simulink model "Simulations"  (R2020b)
settings: Solver=VariableStepAuto  StartTime=0.0  StopTime=100  MinStep=0.0001  RelTol=1e-3
undefined symbols (not defined in the file or in its folder): chassis, FTP, powertrain, sigbuilder_block
libraries: sdl_lib x364, nesl_utility x336, fl_lib x224, aerolibconvert2 x28, pid_lib x27
(part 14 of 15)

== system Simulations/Plant Model7 ==
  note: Chassis
  note: Motor Dynamics
  note: Drivetrain
  trq_cmd : Inport
  road_grade : Inport  Port=2
  Angle Conversion3 : aerolibconvert2/Angle Conversion  IU=deg  OU=rad
  Belt Drive FL : sdl_lib/Couplings & Drives/Belt Drive  drive_type=sdl.enum.wrap_configuration.open  belt_type=sdl.enum.belt_type.ideal  sheave_ang=30 deg  num_belts=1  model_f_c=sdl.enum.model_centrifugal.off  linear_density=0.6 kg/m  model_compliance=sdl.enum.compliance.off  stiffness=1e4 N/m  damping=1e3 N/(m/s)  tension=100 N  breakable=sdl.enum.max_tension.off  F_max=1e5 N  r_pulley_A=drivetrain.RadiusA m  r_pulley_B=drivetrain.RadiusB m  b_pulley_A=drivetrain.bvfCoeffA N*m/(rad/s)  b_pulley_B=drivetrain.bvfCoeffB N*m/(rad/s)  model_inertia_A=sdl.enum.model_inertia.off  model_inertia_B=sdl.enum.model_inertia.off  pulley_inertia_A=0.01 kg*m^2  pulley_inertia_B=0.03 kg*m^2  initial_velocity_A=0 rad/s  initial_velocity_B=0 rad/s  mu=0.5  wrap_parameterization=sdl.enum.wrap_parameterization.centers  d_centers=0.5 m  phi_wrap_A=145 deg  phi_wrap_B=215 deg  v_thr=0.001 m/s
      settings: SourceProductBaseCode=LD  InternalSimscapePortConfiguration="{\"Bottom\":[],\"Left\":[{\"id\":\"A\",\"label\":\"A\",\"type\":\"foundation.mechanical.rotational.rotational\"}],\"Right\":[{\"id\":\"B\",\"label\":\"B\",\"type\":\"foundation.mechanical.rotational.rotational\"}],\"Top\":[]}"
  Belt Drive FR : sdl_lib/Couplings & Drives/Belt Drive  drive_type=sdl.enum.wrap_configuration.open  belt_type=sdl.enum.belt_type.ideal  sheave_ang=30 deg  num_belts=1  model_f_c=sdl.enum.model_centrifugal.off  linear_density=0.6 kg/m  model_compliance=sdl.enum.compliance.off  stiffness=1e4 N/m  damping=1e3 N/(m/s)  tension=100 N  breakable=sdl.enum.max_tension.off  F_max=1e5 N  r_pulley_A=drivetrain.RadiusA m  r_pulley_B=drivetrain.RadiusB m  b_pulley_A=drivetrain.bvfCoeffA N*m/(rad/s)  b_pulley_B=drivetrain.bvfCoeffB N*m/(rad/s)  model_inertia_A=sdl.enum.model_inertia.off  model_inertia_B=sdl.enum.model_inertia.off  pulley_inertia_A=0.01 kg*m^2  pulley_inertia_B=0.03 kg*m^2  initial_velocity_A=0 rad/s  initial_velocity_B=0 rad/s  mu=0.5  wrap_parameterization=sdl.enum.wrap_parameterization.centers  d_centers=0.5 m  phi_wrap_A=145 deg  phi_wrap_B=215 deg  v_thr=0.001 m/s
      settings: SourceProductBaseCode=LD  InternalSimscapePortConfiguration="{\"Bottom\":[],\"Left\":[{\"id\":\"A\",\"label\":\"A\",\"type\":\"foundation.mechanical.rotational.rotational\"}],\"Right\":[{\"id\":\"B\",\"label\":\"B\",\"type\":\"foundation.mechanical.rotational.rotational\"}],\"Top\":[]}"
  Belt Drive RL : sdl_lib/Couplings & Drives/Belt Drive  drive_type=sdl.enum.wrap_configuration.open  belt_type=sdl.enum.belt_type.ideal  sheave_ang=30 deg  num_belts=1  model_f_c=sdl.enum.model_centrifugal.off  linear_density=0.6 kg/m  model_compliance=sdl.enum.compliance.off  stiffness=1e4 N/m  damping=1e3 N/(m/s)  tension=100 N  breakable=sdl.enum.max_tension.off  F_max=1e5 N  r_pulley_A=drivetrain.RadiusA m  r_pulley_B=drivetrain.RadiusB m  b_pulley_A=drivetrain.bvfCoeffA N*m/(rad/s)  b_pulley_B=drivetrain.bvfCoeffB N*m/(rad/s)  model_inertia_A=sdl.enum.model_inertia.off  model_inertia_B=sdl.enum.model_inertia.off  pulley_inertia_A=0.01 kg*m^2  pulley_inertia_B=0.03 kg*m^2  initial_velocity_A=0 rad/s  initial_velocity_B=0 rad/s  mu=0.5  wrap_parameterization=sdl.enum.wrap_parameterization.centers  d_centers=0.5 m  phi_wrap_A=145 deg  phi_wrap_B=215 deg  v_thr=0.001 m/s
      settings: SourceProductBaseCode=LD  InternalSimscapePortConfiguration="{\"Bottom\":[],\"Left\":[{\"id\":\"A\",\"label\":\"A\",\"type\":\"foundation.mechanical.rotational.rotational\"}],\"Right\":[{\"id\":\"B\",\"label\":\"B\",\"type\":\"foundation.mechanical.rotational.rotational\"}],\"Top\":[]}"
  Belt Drive RR : sdl_lib/Couplings & Drives/Belt Drive  drive_type=sdl.enum.wrap_configuration.open  belt_type=sdl.enum.belt_type.ideal  sheave_ang=30 deg  num_belts=1  model_f_c=sdl.enum.model_centrifugal.off  linear_density=0.6 kg/m  model_compliance=sdl.enum.compliance.off  stiffness=1e4 N/m  damping=1e3 N/(m/s)  tension=100 N  breakable=sdl.enum.max_tension.off  F_max=1e5 N  r_pulley_A=drivetrain.RadiusA m  r_pulley_B=drivetrain.RadiusB m  b_pulley_A=drivetrain.bvfCoeffA N*m/(rad/s)  b_pulley_B=drivetrain.bvfCoeffB N*m/(rad/s)  model_inertia_A=sdl.enum.model_inertia.off  model_inertia_B=sdl.enum.model_inertia.off  pulley_inertia_A=0.01 kg*m^2  pulley_inertia_B=0.03 kg*m^2  initial_velocity_A=0 rad/s  initial_velocity_B=0 rad/s  mu=0.5  wrap_parameterization=sdl.enum.wrap_parameterization.centers  d_centers=0.5 m  phi_wrap_A=145 deg  phi_wrap_B=215 deg  v_thr=0.001 m/s
      settings: SourceProductBaseCode=LD  InternalSimscapePortConfiguration="{\"Bottom\":[],\"Left\":[{\"id\":\"A\",\"label\":\"A\",\"type\":\"foundation.mechanical.rotational.rotational\"}],\"Right\":[{\"id\":\"B\",\"label\":\"B\",\"type\":\"foundation.mechanical.rotational.rotational\"}],\"Top\":[]}"
  Constant : Constant  Value=0
  Ideal Torque Source FL : fl_lib/Mechanical/Mechanical Sources/Ideal Torque Source
  Ideal Torque Source FR : fl_lib/Mechanical/Mechanical Sources/Ideal Torque Source
  Ideal Torque Source RL : fl_lib/Mechanical/Mechanical Sources/Ideal Torque Source
  Ideal Torque Source RR : fl_lib/Mechanical/Mechanical Sources/Ideal Torque Source
  Mechanical Rotational Reference{1..3,8} (4 alike) : fl_lib/Mechanical/Rotational Elements/Mechanical Rotational Reference
  Motor Delay : TransferFcn  Numerator=[0.01]  Denominator=[0.005 0.06 0.1001]
  PS-Simulink Converter{,1,3..4} (4 alike) : nesl_utility/PS-Simulink Converter  PhysicalDomain=network_engine_domain  SubClassName=ps_output  LeftPortType=input  RightPortType=output  PseudoPeriodic=off  Frequencies=[]  Unit=inherit  AffineConversion=off
  Simulink-PS Converter{3,9..12} (5 alike) : nesl_utility/Simulink-PS Converter  PhysicalDomain=network_engine_domain  SubClassName=ps_input  LeftPortType=input  RightPortType=output  PseudoPeriodic=off  Frequencies=[]  NoiseDistribution=none  NoiseParameters=[]  Unit=1  AffineConversion=off  FilteringAndDerivatives=provide  SimscapeFilterOrder=1  InputFilterTimeConstant=0.001  UdotUserProvided=0
  Simulink-PS Converter8 : nesl_utility/Simulink-PS Converter  PhysicalDomain=network_engine_domain  SubClassName=ps_input  LeftPortType=input  RightPortType=output  PseudoPeriodic=off  Frequencies=[]  NoiseDistribution=none  NoiseParameters=[]  Unit=rad  AffineConversion=off  FilteringAndDerivatives=provide  SimscapeFilterOrder=1  InputFilterTimeConstant=0.001  UdotUserProvided=0
  Solver Configuration2 : nesl_utility/Solver Configuration  PhysicalDomain=network_engine_domain  SubClassName=solver  LeftPortType=input  RightPortType=generic  Tones=[]  Harmonics=[]  SimulateNoise=off  Profile=off  UseLocalSampling=off  EnableSwitchedLinearOptims=on  FrequencyDomain=off  UseCCode=off  RelTol=0.001  AbsTol=1e-06  MinStep=1e-09  ToWorkspace=off  RevertToSquareIcSolve=off  NumHomotopyIterations=100  PhasorMode=off  PhasorModeNumHarmonics=1  DoDC=off  ResidualTolerance=1e-09  UseLocalSolver=off  LocalSolverChoice=NE_BACKWARD_EULER_ADVANCER  LocalSolverSampleTime=0.001  DoFixedCost=off  MaxNonlinIter=3  MaxModeIter=2  ComputeImpulses=off  ImpulseIterations=2  LinearAlgebra=auto  EquationFormulation=NE_TIME_EF  DelaysMemoryBudget=1024  AutomaticFiltering=on  FilteringTimeConstant=0.001  PartitionStorageMethod=AS_NEEDED  PartitionMemoryBudget=1024  PartitionMethod=ROBUST
  Terminator{,1..3} (4 alike) : Terminator
  Tire (Simple) FL : sdl_lib/Tires & Vehicles/Tire (Simple)  r_tire=drivetrain.RolRadius m  model_compliance=0  stiffness=1e6 N/m  damping=1000 N/(m/s)  model_inertia=0  tire_inertia=drivetrain.IyyWhl kg*m^2  initial_velocity=drivetrain.InitVelo rad/s
      settings: SourceProductBaseCode=LD  InternalSimscapePortConfiguration="{\"Bottom\":[],\"Left\":[{\"id\":\"A\",\"label\":\"A\",\"type\":\"foundation.mechanical.rotational.rotational\"}],\"Right\":[{\"id\":\"H\",\"label\":\"H\",\"type\":\"foundation.mechanical.translational.translational\"}],\"Top\":[]}"
  Tire (Simple) FR : sdl_lib/Tires & Vehicles/Tire (Simple)  r_tire=drivetrain.RolRadius m  model_compliance=0  stiffness=1e6 N/m  damping=1000 N/(m/s)  model_inertia=0  tire_inertia=drivetrain.IyyWhl kg*m^2  initial_velocity=drivetrain.InitVelo rad/s
      settings: SourceProductBaseCode=LD  InternalSimscapePortConfiguration="{\"Bottom\":[],\"Left\":[{\"id\":\"A\",\"label\":\"A\",\"type\":\"foundation.mechanical.rotational.rotational\"}],\"Right\":[{\"id\":\"H\",\"label\":\"H\",\"type\":\"foundation.mechanical.translational.translational\"}],\"Top\":[]}"
  Tire (Simple) RL : sdl_lib/Tires & Vehicles/Tire (Simple)  r_tire=drivetrain.RolRadius m  model_compliance=0  stiffness=1e6 N/m  damping=1000 N/(m/s)  model_inertia=0  tire_inertia=drivetrain.IyyWhl kg*m^2  initial_velocity=drivetrain.InitVelo rad/s
      settings: SourceProductBaseCode=LD  InternalSimscapePortConfiguration="{\"Bottom\":[],\"Left\":[{\"id\":\"A\",\"label\":\"A\",\"type\":\"foundation.mechanical.rotational.rotational\"}],\"Right\":[{\"id\":\"H\",\"label\":\"H\",\"type\":\"foundation.mechanical.translational.translational\"}],\"Top\":[]}"
  Tire (Simple) RR : sdl_lib/Tires & Vehicles/Tire (Simple)  r_tire=drivetrain.RolRadius m  model_compliance=0  stiffness=1e6 N/m  damping=1000 N/(m/s)  model_inertia=0  tire_inertia=drivetrain.IyyWhl kg*m^2  initial_velocity=drivetrain.InitVelo rad/s
      settings: SourceProductBaseCode=LD  InternalSimscapePortConfiguration="{\"Bottom\":[],\"Left\":[{\"id\":\"A\",\"label\":\"A\",\"type\":\"foundation.mechanical.rotational.rotational\"}],\"Right\":[{\"id\":\"H\",\"label\":\"H\",\"type\":\"foundation.mechanical.translational.translational\"}],\"Top\":[]}"
  Tire-Road Interaction (Magic Formula) FL : sdl_lib/Tires & Vehicles/Tire Subcomponents/Tire-Road Interaction (Magic Formula)  parameterization=sdl.enum.magic_tire_model.peak  F_z1=drivetrain.VertLoad N  F_x1=drivetrain.PeakLongF N  kappa1=drivetrain.Slip  B_m=10  C_m=1.9  D_m=1  E_m=0.97  fz0=4000 N  p_Cx=1.685  p_Dx=[1.21, -.037]  p_Ex=[.344, .095, -.02, 0]  p_Kx=[21.51, -.163, .245]  p_Hx=[-.002, .002]  p_Vx=[0, 0]  v_tr_thr=drivetrain.VeloTrhd m/s
      settings: SourceProductBaseCode=LD  InternalSimscapePortConfiguration="{\"Bottom\":[],\"Left\":[{\"id\":\"N\",\"label\":\"N\",\"type\":\"input\"},{\"id\":\"T\",\"label\":\"T\",\"type\":\"foundation.mechanical.translational.translational\"}],\"Right\":[{\"id\":\"S\",\"label\":\"S\",\"type\":\"output\"},{\"id\":\"H\",\"label\":\"H\",\"type\":\"foundation.mechanical.translational.translational\"}],\"Top\":[]}"
  Tire-Road Interaction (Magic Formula) FR : sdl_lib/Tires & Vehicles/Tire Subcomponents/Tire-Road Interaction (Magic Formula)  parameterization=sdl.enum.magic_tire_model.peak  F_z1=drivetrain.VertLoad N  F_x1=drivetrain.PeakLongF N  kappa1=drivetrain.Slip  B_m=10  C_m=1.9  D_m=1  E_m=0.97  fz0=4000 N  p_Cx=1.685  p_Dx=[1.21, -.037]  p_Ex=[.344, .095, -.02, 0]  p_Kx=[21.51, -.163, .245]  p_Hx=[-.002, .002]  p_Vx=[0, 0]  v_tr_thr=drivetrain.VeloTrhd m/s
      settings: SourceProductBaseCode=LD  InternalSimscapePortConfiguration="{\"Bottom\":[],\"Left\":[{\"id\":\"N\",\"label\":\"N\",\"type\":\"input\"},{\"id\":\"T\",\"label\":\"T\",\"type\":\"foundation.mechanical.translational.translational\"}],\"Right\":[{\"id\":\"S\",\"label\":\"S\",\"type\":\"output\"},{\"id\":\"H\",\"label\":\"H\",\"type\":\"foundation.mechanical.translational.translational\"}],\"Top\":[]}"
  Tire-Road Interaction (Magic Formula) RL : sdl_lib/Tires & Vehicles/Tire Subcomponents/Tire-Road Interaction (Magic Formula)  parameterization=sdl.enum.magic_tire_model.peak  F_z1=drivetrain.VertLoad N  F_x1=drivetrain.PeakLongF N  kappa1=drivetrain.Slip  B_m=10  C_m=1.9  D_m=1  E_m=0.97  fz0=4000 N  p_Cx=1.685  p_Dx=[1.21, -.037]  p_Ex=[.344, .095, -.02, 0]  p_Kx=[21.51, -.163, .245]  p_Hx=[-.002, .002]  p_Vx=[0, 0]  v_tr_thr=drivetrain.VeloTrhd m/s
      settings: SourceProductBaseCode=LD  InternalSimscapePortConfiguration="{\"Bottom\":[],\"Left\":[{\"id\":\"N\",\"label\":\"N\",\"type\":\"input\"},{\"id\":\"T\",\"label\":\"T\",\"type\":\"foundation.mechanical.translational.translational\"}],\"Right\":[{\"id\":\"S\",\"label\":\"S\",\"type\":\"output\"},{\"id\":\"H\",\"label\":\"H\",\"type\":\"foundation.mechanical.translational.translational\"}],\"Top\":[]}"
  Tire-Road Interaction (Magic Formula) RR : sdl_lib/Tires & Vehicles/Tire Subcomponents/Tire-Road Interaction (Magic Formula)  parameterization=sdl.enum.magic_tire_model.peak  F_z1=drivetrain.VertLoad N  F_x1=drivetrain.PeakLongF N  kappa1=drivetrain.Slip  B_m=10  C_m=1.9  D_m=1  E_m=0.97  fz0=4000 N  p_Cx=1.685  p_Dx=[1.21, -.037]  p_Ex=[.344, .095, -.02, 0]  p_Kx=[21.51, -.163, .245]  p_Hx=[-.002, .002]  p_Vx=[0, 0]  v_tr_thr=drivetrain.VeloTrhd m/s
      settings: SourceProductBaseCode=LD  InternalSimscapePortConfiguration="{\"Bottom\":[],\"Left\":[{\"id\":\"N\",\"label\":\"N\",\"type\":\"input\"},{\"id\":\"T\",\"label\":\"T\",\"type\":\"foundation.mechanical.translational.translational\"}],\"Right\":[{\"id\":\"S\",\"label\":\"S\",\"type\":\"output\"},{\"id\":\"H\",\"label\":\"H\",\"type\":\"foundation.mechanical.translational.translational\"}],\"Top\":[]}"
  Vehicle Body : sdl_lib/Tires & Vehicles/Vehicle Body  mass=chassis.m kg  n_w=chassis.NumWhl  x_f=chassis.a m  x_r=chassis.b m  y_c="chassis.h  m"  mass_var=simscape.enum.onoff.off  model_pitch=simscape.enum.onoff.off  inertia=4000 kg*m^2  suspension_model=sdl.enum.linearTLU.linear  k_f=1e4 N/m  b_f=1e4 N/(m/s)  k_r=1e4 N/m  b_r=1e4 N/(m/s)  k_f_TLU=[-2000, -1000, 0, 1000, 2000] N  x_f_TLU=[-.4, -.2, 0, .2, .4] m  b_f_TLU=[-200, -100, 0, 100, 200] N  v_f_TLU=[-4, -2, 0, 2, 4] m/s  k_r_TLU=[-2000, -1000, 0, 1000, 2000] N  x_r_TLU=[-.4, -.2, 0, .2, .4] m  b_r_TLU=[-200, -100, 0, 100, 200] N  v_r_TLU=[-4, -2, 0, 2, 4] m/s  interp_method=simscape.enum.interpolation.linear  extrap_method=simscape.enum.extrapolation.linear  model_hardstop=simscape.enum.onoff.off  upper_bound_f=.25 m  lower_bound_f=-.25 m  stop_k_f=1e6 N/m  stop_b_f=150 N/(m/s)  upper_bound_r=.25 m  lower_bound_r=-.25 m  stop_k_r=1e6 N/m  stop_b_r=150 N/(m/s)  initial_pitch=0 rad  initial_pitch_rate=0 rad/s  g=chassis.g m/s^2  liftoff_warning=simscape.enum.onoff.off  area=chassis.Af m^2  Cd=chassis.Cd  rho=chassis.AirDensity kg/m^3  v_specify=off  v_priority=High  v=0 m/s  v_nominal_specify=off  v_nominal_unit=m/s  v_nominal_value=1
  v_lin1 : nesl_utility/PS-Simulink Converter  PhysicalDomain=network_engine_domain  SubClassName=ps_output  LeftPortType=input  RightPortType=output  PseudoPeriodic=off  Frequencies=[]  Unit=inherit  AffineConversion=off
  veh_spd_lin : Outport
  wires:
  Motor Delay/1 -> Simulink-PS Converter9/1, Simulink-PS Converter11/1, Simulink-PS Converter12/1, Simulink-PS Converter10/1  "trq_act_PID"
  v_lin1/1 -> veh_spd_lin/1  "act"
  PS-Simulink Converter/1 -> Terminator/1
  PS-Simulink Converter1/1 -> Terminator1/1
  PS-Simulink Converter3/1 -> Terminator2/1
  PS-Simulink Converter4/1 -> Terminator3/1
  trq_cmd/1 -> Motor Delay/1  "trq_act_before_delay_PID"
  road_grade/1 -> Angle Conversion3/1
  Angle Conversion3/1 -> Simulink-PS Converter8/1
  Constant/1 -> Simulink-PS Converter3/1
  connections:
  Vehicle Body/RConn2 -- Tire-Road Interaction (Magic Formula) FR/LConn1 -- Tire-Road Interaction (Magic Formula) FL/LConn1
  Vehicle Body/LConn1 -- Tire-Road Interaction (Magic Formula) RR/RConn2 -- Tire-Road Interaction (Magic Formula) RL/RConn2 -- Tire-Road Interaction (Magic Formula) FR/RConn2 -- Tire-Road Interaction (Magic Formula) FL/RConn2
  Solver Configuration2/RConn1 -- Simulink-PS Converter9/RConn1 -- Ideal Torque Source RR/RConn1
  Vehicle Body/RConn1 -- Tire-Road Interaction (Magic Formula) RR/LConn1 -- Tire-Road Interaction (Magic Formula) RL/LConn1
  Belt Drive FR/RConn1 -- Tire (Simple) FR/LConn1
  Simulink-PS Converter10/RConn1 -- Ideal Torque Source RL/RConn1
  Simulink-PS Converter12/RConn1 -- Ideal Torque Source FL/RConn1
  Tire (Simple) RL/RConn1 -- Tire-Road Interaction (Magic Formula) RL/LConn2
  Simulink-PS Converter11/RConn1 -- Ideal Torque Source FR/RConn1
  Belt Drive FR/LConn1 -- Ideal Torque Source FR/LConn1
  Belt Drive RL/LConn1 -- Ideal Torque Source RL/LConn1
  Mechanical Rotational Reference3/LConn1 -- Ideal Torque Source FR/RConn2
  Belt Drive RR/RConn1 -- Tire (Simple) RR/LConn1
  Belt Drive FL/RConn1 -- Tire (Simple) FL/LConn1
  Mechanical Rotational Reference1/LConn1 -- Ideal Torque Source RR/RConn2
  v_lin1/LConn1 -- Vehicle Body/LConn2
  Belt Drive RL/RConn1 -- Tire (Simple) RL/LConn1
  Tire (Simple) FR/RConn1 -- Tire-Road Interaction (Magic Formula) FR/LConn2
  Vehicle Body/RConn3 -- Simulink-PS Converter8/RConn1
  Mechanical Rotational Reference8/LConn1 -- Ideal Torque Source FL/RConn2
  Simulink-PS Converter3/RConn1 -- Vehicle Body/LConn3
  Tire (Simple) RR/RConn1 -- Tire-Road Interaction (Magic Formula) RR/LConn2
  Tire (Simple) FL/RConn1 -- Tire-Road Interaction (Magic Formula) FL/LConn2
  Mechanical Rotational Reference2/LConn1 -- Ideal Torque Source RL/RConn2
  Belt Drive RR/LConn1 -- Ideal Torque Source RR/LConn1
  Belt Drive FL/LConn1 -- Ideal Torque Source FL/LConn1
  Tire-Road Interaction (Magic Formula) RR/RConn1 -- PS-Simulink Converter/LConn1
  PS-Simulink Converter1/LConn1 -- Tire-Road Interaction (Magic Formula) RL/RConn1
  PS-Simulink Converter3/LConn1 -- Tire-Road Interaction (Magic Formula) FR/RConn1
  PS-Simulink Converter4/LConn1 -- Tire-Road Interaction (Magic Formula) FL/RConn1

== system Simulations/Plant Model8 ==
  note: Chassis
  note: Motor Dynamics
  note: Drivetrain
  trq_cmd : Inport
  road_grade : Inport  Port=2
  Angle Conversion3 : aerolibconvert2/Angle Conversion  IU=deg  OU=rad
  Belt Drive FL : sdl_lib/Couplings & Drives/Belt Drive  drive_type=sdl.enum.wrap_configuration.open  belt_type=sdl.enum.belt_type.ideal  sheave_ang=30 deg  num_belts=1  model_f_c=sdl.enum.model_centrifugal.off  linear_density=0.6 kg/m  model_compliance=sdl.enum.compliance.off  stiffness=1e4 N/m  damping=1e3 N/(m/s)  tension=100 N  breakable=sdl.enum.max_tension.off  F_max=1e5 N  r_pulley_A=drivetrain.RadiusA m  r_pulley_B=drivetrain.RadiusB m  b_pulley_A=drivetrain.bvfCoeffA N*m/(rad/s)  b_pulley_B=drivetrain.bvfCoeffB N*m/(rad/s)  model_inertia_A=sdl.enum.model_inertia.off  model_inertia_B=sdl.enum.model_inertia.off  pulley_inertia_A=0.01 kg*m^2  pulley_inertia_B=0.03 kg*m^2  initial_velocity_A=0 rad/s  initial_velocity_B=0 rad/s  mu=0.5  wrap_parameterization=sdl.enum.wrap_parameterization.centers  d_centers=0.5 m  phi_wrap_A=145 deg  phi_wrap_B=215 deg  v_thr=0.001 m/s
      settings: SourceProductBaseCode=LD  InternalSimscapePortConfiguration="{\"Bottom\":[],\"Left\":[{\"id\":\"A\",\"label\":\"A\",\"type\":\"foundation.mechanical.rotational.rotational\"}],\"Right\":[{\"id\":\"B\",\"label\":\"B\",\"type\":\"foundation.mechanical.rotational.rotational\"}],\"Top\":[]}"
  Belt Drive FR : sdl_lib/Couplings & Drives/Belt Drive  drive_type=sdl.enum.wrap_configuration.open  belt_type=sdl.enum.belt_type.ideal  sheave_ang=30 deg  num_belts=1  model_f_c=sdl.enum.model_centrifugal.off  linear_density=0.6 kg/m  model_compliance=sdl.enum.compliance.off  stiffness=1e4 N/m  damping=1e3 N/(m/s)  tension=100 N  breakable=sdl.enum.max_tension.off  F_max=1e5 N  r_pulley_A=drivetrain.RadiusA m  r_pulley_B=drivetrain.RadiusB m  b_pulley_A=drivetrain.bvfCoeffA N*m/(rad/s)  b_pulley_B=drivetrain.bvfCoeffB N*m/(rad/s)  model_inertia_A=sdl.enum.model_inertia.off  model_inertia_B=sdl.enum.model_inertia.off  pulley_inertia_A=0.01 kg*m^2  pulley_inertia_B=0.03 kg*m^2  initial_velocity_A=0 rad/s  initial_velocity_B=0 rad/s  mu=0.5  wrap_parameterization=sdl.enum.wrap_parameterization.centers  d_centers=0.5 m  phi_wrap_A=145 deg  phi_wrap_B=215 deg  v_thr=0.001 m/s
      settings: SourceProductBaseCode=LD  InternalSimscapePortConfiguration="{\"Bottom\":[],\"Left\":[{\"id\":\"A\",\"label\":\"A\",\"type\":\"foundation.mechanical.rotational.rotational\"}],\"Right\":[{\"id\":\"B\",\"label\":\"B\",\"type\":\"foundation.mechanical.rotational.rotational\"}],\"Top\":[]}"
  Belt Drive RL : sdl_lib/Couplings & Drives/Belt Drive  drive_type=sdl.enum.wrap_configuration.open  belt_type=sdl.enum.belt_type.ideal  sheave_ang=30 deg  num_belts=1  model_f_c=sdl.enum.model_centrifugal.off  linear_density=0.6 kg/m  model_compliance=sdl.enum.compliance.off  stiffness=1e4 N/m  damping=1e3 N/(m/s)  tension=100 N  breakable=sdl.enum.max_tension.off  F_max=1e5 N  r_pulley_A=drivetrain.RadiusA m  r_pulley_B=drivetrain.RadiusB m  b_pulley_A=drivetrain.bvfCoeffA N*m/(rad/s)  b_pulley_B=drivetrain.bvfCoeffB N*m/(rad/s)  model_inertia_A=sdl.enum.model_inertia.off  model_inertia_B=sdl.enum.model_inertia.off  pulley_inertia_A=0.01 kg*m^2  pulley_inertia_B=0.03 kg*m^2  initial_velocity_A=0 rad/s  initial_velocity_B=0 rad/s  mu=0.5  wrap_parameterization=sdl.enum.wrap_parameterization.centers  d_centers=0.5 m  phi_wrap_A=145 deg  phi_wrap_B=215 deg  v_thr=0.001 m/s
      settings: SourceProductBaseCode=LD  InternalSimscapePortConfiguration="{\"Bottom\":[],\"Left\":[{\"id\":\"A\",\"label\":\"A\",\"type\":\"foundation.mechanical.rotational.rotational\"}],\"Right\":[{\"id\":\"B\",\"label\":\"B\",\"type\":\"foundation.mechanical.rotational.rotational\"}],\"Top\":[]}"
  Belt Drive RR : sdl_lib/Couplings & Drives/Belt Drive  drive_type=sdl.enum.wrap_configuration.open  belt_type=sdl.enum.belt_type.ideal  sheave_ang=30 deg  num_belts=1  model_f_c=sdl.enum.model_centrifugal.off  linear_density=0.6 kg/m  model_compliance=sdl.enum.compliance.off  stiffness=1e4 N/m  damping=1e3 N/(m/s)  tension=100 N  breakable=sdl.enum.max_tension.off  F_max=1e5 N  r_pulley_A=drivetrain.RadiusA m  r_pulley_B=drivetrain.RadiusB m  b_pulley_A=drivetrain.bvfCoeffA N*m/(rad/s)  b_pulley_B=drivetrain.bvfCoeffB N*m/(rad/s)  model_inertia_A=sdl.enum.model_inertia.off  model_inertia_B=sdl.enum.model_inertia.off  pulley_inertia_A=0.01 kg*m^2  pulley_inertia_B=0.03 kg*m^2  initial_velocity_A=0 rad/s  initial_velocity_B=0 rad/s  mu=0.5  wrap_parameterization=sdl.enum.wrap_parameterization.centers  d_centers=0.5 m  phi_wrap_A=145 deg  phi_wrap_B=215 deg  v_thr=0.001 m/s
      settings: SourceProductBaseCode=LD  InternalSimscapePortConfiguration="{\"Bottom\":[],\"Left\":[{\"id\":\"A\",\"label\":\"A\",\"type\":\"foundation.mechanical.rotational.rotational\"}],\"Right\":[{\"id\":\"B\",\"label\":\"B\",\"type\":\"foundation.mechanical.rotational.rotational\"}],\"Top\":[]}"
  Constant : Constant  Value=0
  Ideal Torque Source FL : fl_lib/Mechanical/Mechanical Sources/Ideal Torque Source
  Ideal Torque Source FR : fl_lib/Mechanical/Mechanical Sources/Ideal Torque Source
  Ideal Torque Source RL : fl_lib/Mechanical/Mechanical Sources/Ideal Torque Source
  Ideal Torque Source RR : fl_lib/Mechanical/Mechanical Sources/Ideal Torque Source
  Mechanical Rotational Reference{1..3,8} (4 alike) : fl_lib/Mechanical/Rotational Elements/Mechanical Rotational Reference
  Motor Delay : TransferFcn  Numerator=[0.01]  Denominator=[0.005 0.06 0.1001]
  PS-Simulink Converter{,1,3..4} (4 alike) : nesl_utility/PS-Simulink Converter  PhysicalDomain=network_engine_domain  SubClassName=ps_output  LeftPortType=input  RightPortType=output  PseudoPeriodic=off  Frequencies=[]  Unit=inherit  AffineConversion=off
  Simulink-PS Converter{3,9..12} (5 alike) : nesl_utility/Simulink-PS Converter  PhysicalDomain=network_engine_domain  SubClassName=ps_input  LeftPortType=input  RightPortType=output  PseudoPeriodic=off  Frequencies=[]  NoiseDistribution=none  NoiseParameters=[]  Unit=1  AffineConversion=off  FilteringAndDerivatives=provide  SimscapeFilterOrder=1  InputFilterTimeConstant=0.001  UdotUserProvided=0
  Simulink-PS Converter8 : nesl_utility/Simulink-PS Converter  PhysicalDomain=network_engine_domain  SubClassName=ps_input  LeftPortType=input  RightPortType=output  PseudoPeriodic=off  Frequencies=[]  NoiseDistribution=none  NoiseParameters=[]  Unit=rad  AffineConversion=off  FilteringAndDerivatives=provide  SimscapeFilterOrder=1  InputFilterTimeConstant=0.001  UdotUserProvided=0
  Solver Configuration2 : nesl_utility/Solver Configuration  PhysicalDomain=network_engine_domain  SubClassName=solver  LeftPortType=input  RightPortType=generic  Tones=[]  Harmonics=[]  SimulateNoise=off  Profile=off  UseLocalSampling=off  EnableSwitchedLinearOptims=on  FrequencyDomain=off  UseCCode=off  RelTol=0.001  AbsTol=1e-06  MinStep=1e-09  ToWorkspace=off  RevertToSquareIcSolve=off  NumHomotopyIterations=100  PhasorMode=off  PhasorModeNumHarmonics=1  DoDC=off  ResidualTolerance=1e-09  UseLocalSolver=off  LocalSolverChoice=NE_BACKWARD_EULER_ADVANCER  LocalSolverSampleTime=0.001  DoFixedCost=off  MaxNonlinIter=3  MaxModeIter=2  ComputeImpulses=off  ImpulseIterations=2  LinearAlgebra=auto  EquationFormulation=NE_TIME_EF  DelaysMemoryBudget=1024  AutomaticFiltering=on  FilteringTimeConstant=0.001  PartitionStorageMethod=AS_NEEDED  PartitionMemoryBudget=1024  PartitionMethod=ROBUST
  Terminator{,1..3} (4 alike) : Terminator
  Tire (Simple) FL : sdl_lib/Tires & Vehicles/Tire (Simple)  r_tire=drivetrain.RolRadius m  model_compliance=0  stiffness=1e6 N/m  damping=1000 N/(m/s)  model_inertia=0  tire_inertia=drivetrain.IyyWhl kg*m^2  initial_velocity=drivetrain.InitVelo rad/s
      settings: SourceProductBaseCode=LD  InternalSimscapePortConfiguration="{\"Bottom\":[],\"Left\":[{\"id\":\"A\",\"label\":\"A\",\"type\":\"foundation.mechanical.rotational.rotational\"}],\"Right\":[{\"id\":\"H\",\"label\":\"H\",\"type\":\"foundation.mechanical.translational.translational\"}],\"Top\":[]}"
  Tire (Simple) FR : sdl_lib/Tires & Vehicles/Tire (Simple)  r_tire=drivetrain.RolRadius m  model_compliance=0  stiffness=1e6 N/m  damping=1000 N/(m/s)  model_inertia=0  tire_inertia=drivetrain.IyyWhl kg*m^2  initial_velocity=drivetrain.InitVelo rad/s
      settings: SourceProductBaseCode=LD  InternalSimscapePortConfiguration="{\"Bottom\":[],\"Left\":[{\"id\":\"A\",\"label\":\"A\",\"type\":\"foundation.mechanical.rotational.rotational\"}],\"Right\":[{\"id\":\"H\",\"label\":\"H\",\"type\":\"foundation.mechanical.translational.translational\"}],\"Top\":[]}"
  Tire (Simple) RL : sdl_lib/Tires & Vehicles/Tire (Simple)  r_tire=drivetrain.RolRadius m  model_compliance=0  stiffness=1e6 N/m  damping=1000 N/(m/s)  model_inertia=0  tire_inertia=drivetrain.IyyWhl kg*m^2  initial_velocity=drivetrain.InitVelo rad/s
      settings: SourceProductBaseCode=LD  InternalSimscapePortConfiguration="{\"Bottom\":[],\"Left\":[{\"id\":\"A\",\"label\":\"A\",\"type\":\"foundation.mechanical.rotational.rotational\"}],\"Right\":[{\"id\":\"H\",\"label\":\"H\",\"type\":\"foundation.mechanical.translational.translational\"}],\"Top\":[]}"
  Tire (Simple) RR : sdl_lib/Tires & Vehicles/Tire (Simple)  r_tire=drivetrain.RolRadius m  model_compliance=0  stiffness=1e6 N/m  damping=1000 N/(m/s)  model_inertia=0  tire_inertia=drivetrain.IyyWhl kg*m^2  initial_velocity=drivetrain.InitVelo rad/s
      settings: SourceProductBaseCode=LD  InternalSimscapePortConfiguration="{\"Bottom\":[],\"Left\":[{\"id\":\"A\",\"label\":\"A\",\"type\":\"foundation.mechanical.rotational.rotational\"}],\"Right\":[{\"id\":\"H\",\"label\":\"H\",\"type\":\"foundation.mechanical.translational.translational\"}],\"Top\":[]}"
  Tire-Road Interaction (Magic Formula) FL : sdl_lib/Tires & Vehicles/Tire Subcomponents/Tire-Road Interaction (Magic Formula)  parameterization=sdl.enum.magic_tire_model.peak  F_z1=drivetrain.VertLoad N  F_x1=drivetrain.PeakLongF N  kappa1=drivetrain.Slip  B_m=10  C_m=1.9  D_m=1  E_m=0.97  fz0=4000 N  p_Cx=1.685  p_Dx=[1.21, -.037]  p_Ex=[.344, .095, -.02, 0]  p_Kx=[21.51, -.163, .245]  p_Hx=[-.002, .002]  p_Vx=[0, 0]  v_tr_thr=drivetrain.VeloTrhd m/s
      settings: SourceProductBaseCode=LD  InternalSimscapePortConfiguration="{\"Bottom\":[],\"Left\":[{\"id\":\"N\",\"label\":\"N\",\"type\":\"input\"},{\"id\":\"T\",\"label\":\"T\",\"type\":\"foundation.mechanical.translational.translational\"}],\"Right\":[{\"id\":\"S\",\"label\":\"S\",\"type\":\"output\"},{\"id\":\"H\",\"label\":\"H\",\"type\":\"foundation.mechanical.translational.translational\"}],\"Top\":[]}"
  Tire-Road Interaction (Magic Formula) FR : sdl_lib/Tires & Vehicles/Tire Subcomponents/Tire-Road Interaction (Magic Formula)  parameterization=sdl.enum.magic_tire_model.peak  F_z1=drivetrain.VertLoad N  F_x1=drivetrain.PeakLongF N  kappa1=drivetrain.Slip  B_m=10  C_m=1.9  D_m=1  E_m=0.97  fz0=4000 N  p_Cx=1.685  p_Dx=[1.21, -.037]  p_Ex=[.344, .095, -.02, 0]  p_Kx=[21.51, -.163, .245]  p_Hx=[-.002, .002]  p_Vx=[0, 0]  v_tr_thr=drivetrain.VeloTrhd m/s
      settings: SourceProductBaseCode=LD  InternalSimscapePortConfiguration="{\"Bottom\":[],\"Left\":[{\"id\":\"N\",\"label\":\"N\",\"type\":\"input\"},{\"id\":\"T\",\"label\":\"T\",\"type\":\"foundation.mechanical.translational.translational\"}],\"Right\":[{\"id\":\"S\",\"label\":\"S\",\"type\":\"output\"},{\"id\":\"H\",\"label\":\"H\",\"type\":\"foundation.mechanical.translational.translational\"}],\"Top\":[]}"
  Tire-Road Interaction (Magic Formula) RL : sdl_lib/Tires & Vehicles/Tire Subcomponents/Tire-Road Interaction (Magic Formula)  parameterization=sdl.enum.magic_tire_model.peak  F_z1=drivetrain.VertLoad N  F_x1=drivetrain.PeakLongF N  kappa1=drivetrain.Slip  B_m=10  C_m=1.9  D_m=1  E_m=0.97  fz0=4000 N  p_Cx=1.685  p_Dx=[1.21, -.037]  p_Ex=[.344, .095, -.02, 0]  p_Kx=[21.51, -.163, .245]  p_Hx=[-.002, .002]  p_Vx=[0, 0]  v_tr_thr=drivetrain.VeloTrhd m/s
      settings: SourceProductBaseCode=LD  InternalSimscapePortConfiguration="{\"Bottom\":[],\"Left\":[{\"id\":\"N\",\"label\":\"N\",\"type\":\"input\"},{\"id\":\"T\",\"label\":\"T\",\"type\":\"foundation.mechanical.translational.translational\"}],\"Right\":[{\"id\":\"S\",\"label\":\"S\",\"type\":\"output\"},{\"id\":\"H\",\"label\":\"H\",\"type\":\"foundation.mechanical.translational.translational\"}],\"Top\":[]}"
  Tire-Road Interaction (Magic Formula) RR : sdl_lib/Tires & Vehicles/Tire Subcomponents/Tire-Road Interaction (Magic Formula)  parameterization=sdl.enum.magic_tire_model.peak  F_z1=drivetrain.VertLoad N  F_x1=drivetrain.PeakLongF N  kappa1=drivetrain.Slip  B_m=10  C_m=1.9  D_m=1  E_m=0.97  fz0=4000 N  p_Cx=1.685  p_Dx=[1.21, -.037]  p_Ex=[.344, .095, -.02, 0]  p_Kx=[21.51, -.163, .245]  p_Hx=[-.002, .002]  p_Vx=[0, 0]  v_tr_thr=drivetrain.VeloTrhd m/s
      settings: SourceProductBaseCode=LD  InternalSimscapePortConfiguration="{\"Bottom\":[],\"Left\":[{\"id\":\"N\",\"label\":\"N\",\"type\":\"input\"},{\"id\":\"T\",\"label\":\"T\",\"type\":\"foundation.mechanical.translational.translational\"}],\"Right\":[{\"id\":\"S\",\"label\":\"S\",\"type\":\"output\"},{\"id\":\"H\",\"label\":\"H\",\"type\":\"foundation.mechanical.translational.translational\"}],\"Top\":[]}"
  Vehicle Body : sdl_lib/Tires & Vehicles/Vehicle Body  mass=chassis.m kg  n_w=chassis.NumWhl  x_f=chassis.a m  x_r=chassis.b m  y_c="chassis.h  m"  mass_var=simscape.enum.onoff.off  model_pitch=simscape.enum.onoff.off  inertia=4000 kg*m^2  suspension_model=sdl.enum.linearTLU.linear  k_f=1e4 N/m  b_f=1e4 N/(m/s)  k_r=1e4 N/m  b_r=1e4 N/(m/s)  k_f_TLU=[-2000, -1000, 0, 1000, 2000] N  x_f_TLU=[-.4, -.2, 0, .2, .4] m  b_f_TLU=[-200, -100, 0, 100, 200] N  v_f_TLU=[-4, -2, 0, 2, 4] m/s  k_r_TLU=[-2000, -1000, 0, 1000, 2000] N  x_r_TLU=[-.4, -.2, 0, .2, .4] m  b_r_TLU=[-200, -100, 0, 100, 200] N  v_r_TLU=[-4, -2, 0, 2, 4] m/s  interp_method=simscape.enum.interpolation.linear  extrap_method=simscape.enum.extrapolation.linear  model_hardstop=simscape.enum.onoff.off  upper_bound_f=.25 m  lower_bound_f=-.25 m  stop_k_f=1e6 N/m  stop_b_f=150 N/(m/s)  upper_bound_r=.25 m  lower_bound_r=-.25 m  stop_k_r=1e6 N/m  stop_b_r=150 N/(m/s)  initial_pitch=0 rad  initial_pitch_rate=0 rad/s  g=chassis.g m/s^2  liftoff_warning=simscape.enum.onoff.off  area=chassis.Af m^2  Cd=chassis.Cd  rho=chassis.AirDensity kg/m^3  v_specify=off  v_priority=High  v=0 m/s  v_nominal_specify=off  v_nominal_unit=m/s  v_nominal_value=1
  v_lin1 : nesl_utility/PS-Simulink Converter  PhysicalDomain=network_engine_domain  SubClassName=ps_output  LeftPortType=input  RightPortType=output  PseudoPeriodic=off  Frequencies=[]  Unit=inherit  AffineConversion=off
  veh_spd_lin : Outport
  wires:
  Motor Delay/1 -> Simulink-PS Converter9/1, Simulink-PS Converter11/1, Simulink-PS Converter12/1, Simulink-PS Converter10/1  "trq_act_PID"
  v_lin1/1 -> veh_spd_lin/1  "act"
  PS-Simulink Converter/1 -> Terminator/1
  PS-Simulink Converter1/1 -> Terminator1/1
  PS-Simulink Converter3/1 -> Terminator2/1
  PS-Simulink Converter4/1 -> Terminator3/1
  trq_cmd/1 -> Motor Delay/1  "trq_act_before_delay_PID"
  road_grade/1 -> Angle Conversion3/1
  Angle Conversion3/1 -> Simulink-PS Converter8/1
  Constant/1 -> Simulink-PS Converter3/1
  connections:
  Vehicle Body/RConn2 -- Tire-Road Interaction (Magic Formula) FR/LConn1 -- Tire-Road Interaction (Magic Formula) FL/LConn1
  Vehicle Body/LConn1 -- Tire-Road Interaction (Magic Formula) RR/RConn2 -- Tire-Road Interaction (Magic Formula) RL/RConn2 -- Tire-Road Interaction (Magic Formula) FR/RConn2 -- Tire-Road Interaction (Magic Formula) FL/RConn2
  Solver Configuration2/RConn1 -- Simulink-PS Converter9/RConn1 -- Ideal Torque Source RR/RConn1
  Vehicle Body/RConn1 -- Tire-Road Interaction (Magic Formula) RR/LConn1 -- Tire-Road Interaction (Magic Formula) RL/LConn1
  Belt Drive FR/RConn1 -- Tire (Simple) FR/LConn1
  Simulink-PS Converter10/RConn1 -- Ideal Torque Source RL/RConn1
  Simulink-PS Converter12/RConn1 -- Ideal Torque Source FL/RConn1
  Tire (Simple) RL/RConn1 -- Tire-Road Interaction (Magic Formula) RL/LConn2
  Simulink-PS Converter11/RConn1 -- Ideal Torque Source FR/RConn1
  Belt Drive FR/LConn1 -- Ideal Torque Source FR/LConn1
  Belt Drive RL/LConn1 -- Ideal Torque Source RL/LConn1
  Mechanical Rotational Reference3/LConn1 -- Ideal Torque Source FR/RConn2
  Belt Drive RR/RConn1 -- Tire (Simple) RR/LConn1
  Belt Drive FL/RConn1 -- Tire (Simple) FL/LConn1
  Mechanical Rotational Reference1/LConn1 -- Ideal Torque Source RR/RConn2
  v_lin1/LConn1 -- Vehicle Body/LConn2
  Belt Drive RL/RConn1 -- Tire (Simple) RL/LConn1
  Tire (Simple) FR/RConn1 -- Tire-Road Interaction (Magic Formula) FR/LConn2
  Vehicle Body/RConn3 -- Simulink-PS Converter8/RConn1
  Mechanical Rotational Reference8/LConn1 -- Ideal Torque Source FL/RConn2
  Simulink-PS Converter3/RConn1 -- Vehicle Body/LConn3
  Tire (Simple) RR/RConn1 -- Tire-Road Interaction (Magic Formula) RR/LConn2
  Tire (Simple) FL/RConn1 -- Tire-Road Interaction (Magic Formula) FL/LConn2
  Mechanical Rotational Reference2/LConn1 -- Ideal Torque Source RL/RConn2
  Belt Drive RR/LConn1 -- Ideal Torque Source RR/LConn1
  Belt Drive FL/LConn1 -- Ideal Torque Source FL/LConn1
  Tire-Road Interaction (Magic Formula) RR/RConn1 -- PS-Simulink Converter/LConn1
  PS-Simulink Converter1/LConn1 -- Tire-Road Interaction (Magic Formula) RL/RConn1
  PS-Simulink Converter3/LConn1 -- Tire-Road Interaction (Magic Formula) FR/RConn1
  PS-Simulink Converter4/LConn1 -- Tire-Road Interaction (Magic Formula) FL/RConn1
